simulink model "pose"  (R2025a)
settings: Solver=VariableStepAuto  StartTime=0.0  StopTime=10.0  RelTol=1e-3
settings Model: Creator=Rudransh  LastModifiedBy=Rudransh

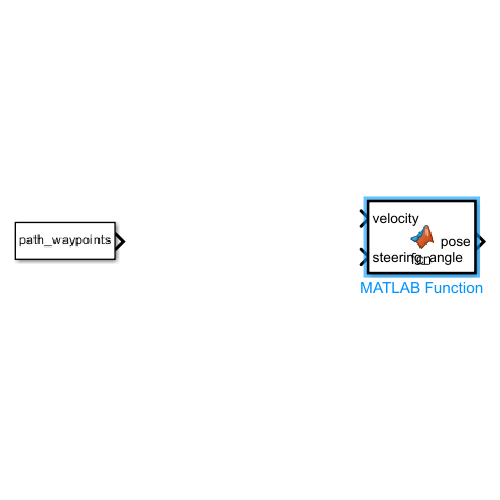
[thumbnail: Simulink's stored preview of the top-level diagram]
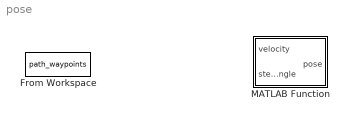
== system pose ==
  From Workspace : FromWorkspace  VariableName=path_waypoints
  MATLAB Function : MATLAB Function  TreatAsAtomicUnit=on

== matlab function pose/MATLAB Function ==
  data: velocity input; pose output; steering_angle input
function pose = VehicleModel(velocity, steering_angle)

% Define vehicle parameters (persistent so they are not reset)
persistent x y theta;

% Initialize vehicle state at the start of the simulation
if isempty(x)
    x = 0;     % Initial x position
    y = 0;     % Initial y position
    theta = 0; % Initial heading angle (radians)
end

% Vehicle constants
L = 2.8; % Wheelbase in meters
Ts = 0.05; % Simulation sample time (must match model's solver)

% Kinematic Bicycle Model equations
x = x + velocity * cos(theta) * Ts;
y = y + velocity * sin(theta) * Ts;
theta = theta + (velocity / L) * tan(steering_angle) * Ts;

% Output the new pose
pose = [x, y, theta];

end
